simulink model "entry_du_ex"  (R2021a)
settings: Solver=FixedStepAuto  StartTime=0.0  StopTime=11.1  FixedStep=1  RelTol=1e-3
settings Model: Creator=surya  LastModifiedBy=surya

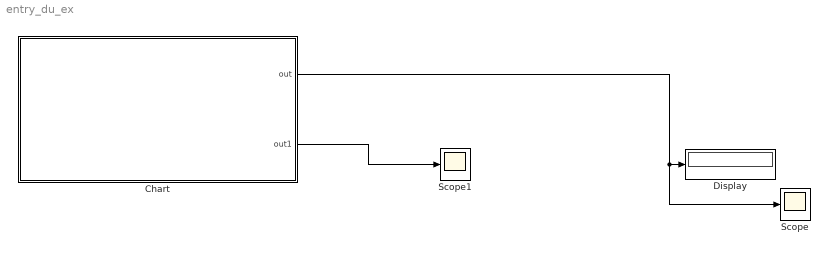
== system entry_du_ex ==
  Chart : Stateflow chart  TreatAsAtomicUnit=on
  Display : Display
  Scope : Scope
  Scope1 : Scope
  wires:
  Chart/1(out) -> Scope/1, Display/1
  Chart/2(out1) -> Scope1/1

== stateflow chart entry_du_ex/Chart ==
  state ON
    en:out=1
    du:out=2;
    ex:out1=3;
  state O
    du:out=5;
    ex:out=6;
  (default) -> ON
  ON -> O
  O -> ON
  data: out output; out1 output
